simulink model "gm_sampleModel61442_pp_12_1_sub"  (R2023b)
settings: Solver=VariableStepAuto  StartTime=0.0  StopTime=10.0  RelTol=1e-3
libraries: simulink x37
(part 1 of 2)
settings Model: Creator=CW  LastModifiedBy=CW
settings OptimizationCC: BlockReduction=off  ConditionallyExecuteInputs=off
settings DebuggingCC: ArtificialAlgebraicLoopMsg=none  InheritedTsInSrcMsg=none

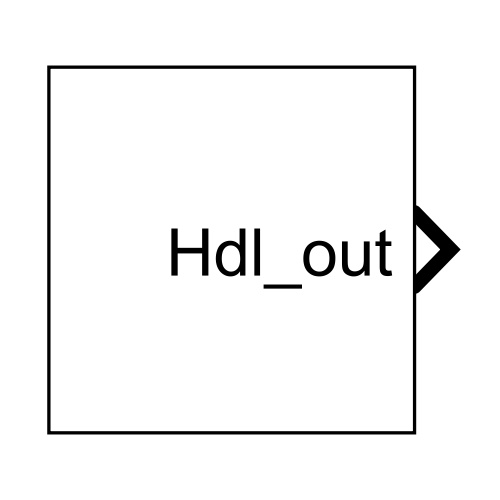
[thumbnail: Simulink's stored preview of the top-level diagram]
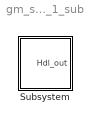
== system gm_sampleModel61442_pp_12_1_sub ==
  Subsystem : Subsystem

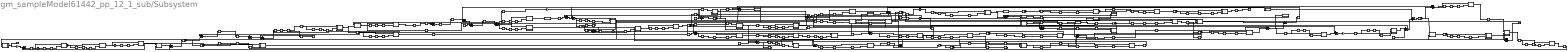
== system gm_sampleModel61442_pp_12_1_sub/Subsystem ==
  Reshape{,1..4} (5 alike) : Reshape
  cfblk1 : Subsystem
  cfblk{10,22,24,46,59,62,66,83,90,93,104} (11 alike) : Sum  Inputs=+  OutDataTypeStr=uint8
  cfblk100 : Subsystem
  cfblk{18,41,50,101} (4 alike) : ComplexToRealImag  SampleTime=1
  cfblk{4..5,14,42,44,57..58,73..74,87,103} (11 alike) : Sum  Inputs=+-  OutDataTypeStr=uint8  AccumDataTypeStr=uint8  SampleTime=1
  cfblk105 : Subsystem
  cfblk106 : Subsystem  mask(Real World Value Increment){}
      mask help: Simulink:masks:RealWorldValueIncrement_MD
      mask Display: disp('V++')
  cfblk108 : Subsystem
  cfblk109 : Subsystem
  cfblk11 : Subsystem
  cfblk110 : Subsystem
  cfblk{26,60,76,96,112} (5 alike) : Gain  Gain="fi(0,0,8,7,\"hex\",\"80\")"  ParamDataTypeStr=fixdt(0, 8, 7)  OutDataTypeStr=uint8  SampleTime=1
  cfblk{68,113,127,129} (4 alike) : MinMax  OutDataTypeStr=uint8
  cfblk{16,27,36,43,51,61,70,82,114..115,118,126,132,142} (14 alike) : Sum  OutDataTypeStr=uint8  AccumDataTypeStr=uint8  SampleTime=1
  cfblk116 : Subsystem
  cfblk{19,30,33,85,117} (5 alike) : Sum  OutDataTypeStr=uint8  AccumDataTypeStr=uint8  RndMeth=Nearest  SampleTime=1
  cfblk117_const_val : Constant  Value=0  VectorParams1D=off  OutDataTypeStr=uint8  SampleTime=1
  cfblk119 : Subsystem
  cfblk{13,35,37,53,64,120,128,138,140} (9 alike) : Abs  SampleTime=1  OutDataTypeStr=uint8  SaturateOnIntegerOverflow=off
  cfblk121 : Subsystem
  cfblk{49,88,99,122,146} (5 alike) : Product  Inputs=*/  OutDataTypeStr=uint8  RndMeth=Zero  SaturateOnIntegerOverflow=on  SampleTime=1
  cfblk{23,39,45,92,98,123,135} (7 alike) : Signum  SampleTime=1
  cfblk124 : Subsystem  mask(Real World Value Increment){}
      mask help: Simulink:masks:RealWorldValueIncrement_MD
      mask Display: disp('V++')
  cfblk125 : Subsystem
  cfblk130_inst : Subsystem
  cfblk134 : Subsystem
  cfblk137 : Subsystem
  cfblk139_inst : Subsystem
  cfblk141_inst : Subsystem
  cfblk143 : Subsystem  mask(Real World Value Increment){}
      mask help: Simulink:masks:RealWorldValueIncrement_MD
      mask Display: disp('V++')
  cfblk144 : Subsystem
  cfblk145 : Subsystem  mask(Real World Value Increment){}
      mask help: Simulink:masks:RealWorldValueIncrement_MD
      mask Display: disp('V++')
  cfblk15 : Subsystem
  cfblk151 : Constant  OutDataTypeStr=uint8  SampleTime=1
  cfblk153 : Subsystem
  cfblk156 : Subsystem
  cfblk157 : Subsystem
  cfblk{158..159,161..167,169..176} (17 alike) : Delay  DelayLength=double(2)  InitialCondition=0  SampleTime=1
  cfblk168 : Subsystem
  cfblk{177..179,182..183,186..187,189..191,193..196} (14 alike) : DataTypeConversion  OutDataTypeStr=fixdt(0,8,0)
  cfblk180 : Subsystem
  cfblk181 : Subsystem
  cfblk184 : Subsystem
  cfblk185 : Subsystem
  cfblk188 : Subsystem
  cfblk192 : Subsystem
  cfblk19_const_val : Constant  Value=0  VectorParams1D=off  OutDataTypeStr=uint8  SampleTime=1
  cfblk2 : Subsystem
  cfblk20 : Subsystem
  cfblk21 : Subsystem
  cfblk25_inst : Subsystem
  cfblk28 : Subsystem
  cfblk3 : Subsystem
  cfblk30_const_val : Constant  Value=0  VectorParams1D=off  OutDataTypeStr=uint8  SampleTime=1
  cfblk31 : Subsystem
  cfblk32 : Subsystem  mask(Real World Value Increment){}
      mask help: Simulink:masks:RealWorldValueIncrement_MD
      mask Display: disp('V++')
  cfblk33_const_val : Constant  Value=0  VectorParams1D=off  OutDataTypeStr=uint8  SampleTime=1
  cfblk40 : Sum  Inputs=+-  OutDataTypeStr=uint8  AccumDataTypeStr=fixdt(1, 32, 7)  SampleTime=1
  cfblk47_inst : Subsystem
  cfblk48 : Subsystem
  cfblk52_inst : Subsystem
  cfblk54_inst : Subsystem
  cfblk71 : Subsystem
  cfblk72 : Subsystem
  cfblk75_inst : Subsystem
  cfblk77 : Subsystem
  cfblk78 : Subsystem
  cfblk79 : Subsystem
  cfblk80 : Subsystem
  cfblk81 : Subsystem
  cfblk84 : Subsystem  mask(Real World Value Increment){}
      mask help: Simulink:masks:RealWorldValueIncrement_MD
      mask Display: disp('V++')
  cfblk85_const_val : Constant  Value=0  VectorParams1D=off  OutDataTypeStr=uint8  SampleTime=1
  cfblk8_inst : Subsystem
  cfblk91 : Subsystem  mask(Real World Value Increment){}
      mask help: Simulink:masks:RealWorldValueIncrement_MD
      mask Display: disp('V++')
  cfblk94_inst : Subsystem
  cfblk97 : Subsystem
  compare{,1,3,7..9,11..15,18..20,22..25,27..28,30,32,35..36} (24 alike) : simulink/Logic and Bit Operations/Compare To Constant  relop=>=  const=0  OutDataTypeStr=boolean
  compare{2,5..6,10,16..17,21,26,29,33} (10 alike) : simulink/Logic and Bit Operations/Compare To Constant  relop=>=  const=255  OutDataTypeStr=boolean
  compare31 : simulink/Logic and Bit Operations/Compare To Constant  relop=>=  const=1  OutDataTypeStr=boolean
  compare34 : simulink/Logic and Bit Operations/Compare To Constant  relop=>=  const=1  OutDataTypeStr=boolean
  compare4 : simulink/Logic and Bit Operations/Compare To Constant  relop=>=  const=1  OutDataTypeStr=boolean
  emi_{6,14,22,30,39,47,55,63,71,79,88,96,104,112,120,128,136,144,152,160,168,176,192,200,208,216,224,232,240,248,256,264,272,281,289,306} (36 alike) : DataTypeConversion  OutDataTypeStr=fixdt(0,8,0)
  emi_{7,23,40,64,89,97,105,113,129,153,161,169,185,193,201,209,233,241,249,265,273,282,290,307} (24 alike) : Delay  DelayLength=double(2)  InitialCondition=0  SampleTime=1
  emi_{31,48,72,121,137,145,177,217,225,257} (10 alike) : Delay  DelayLength=double(2)  InitialCondition=255  SampleTime=1
  emi_15 : Delay  DelayLength=double(2)  InitialCondition=1  SampleTime=1
  emi_184 : DataTypeConversion  OutDataTypeStr=uint8  SampleTime=1  SaturateOnIntegerOverflow=off  RndMeth=Floor
  emi_56 : Delay  DelayLength=double(2)  InitialCondition=1  SampleTime=1
  emi_80 : Delay  DelayLength=double(2)  InitialCondition=1  SampleTime=1
  Hdl_out : Outport  OutDataTypeStr=uint8  SampleTime=1
  wires:
  cfblk1/1(emi_2) -> cfblk60/1, Hdl_out/1
  cfblk10/1 -> emi_129/1, cfblk15/1(emi_123)
  cfblk100/1(emi_10) -> cfblk106/1(u)
  cfblk101/1 -> cfblk146/1
  cfblk101/2 -> cfblk52_inst/1(in1), cfblk187/1
  cfblk103/1 -> cfblk115/2
  cfblk104/1 -> cfblk172/1
  cfblk105/1(emi_18) -> cfblk58/2, cfblk114/1
  cfblk106/1(y) -> cfblk175/1
  cfblk108/1(emi_26) -> emi_225/1, cfblk3/1(emi_219)
  cfblk109/1(emi_34) -> cfblk143/1(u)
  cfblk109/2(emi_35) -> cfblk30/1, cfblk14/1, cfblk170/1
  cfblk11/1(emi_43) -> cfblk101/1
  cfblk110/1(emi_51) -> cfblk40/2
  cfblk112/1 -> cfblk54_inst/2(in2), cfblk10/1
  cfblk113/1 -> cfblk23/1
  cfblk114/1 -> emi_177/1, cfblk21/1(emi_171)
  cfblk115/1 -> cfblk41/1, emi_23/1, cfblk105/1(emi_17)
  cfblk116/1(emi_67) -> cfblk33/1
  cfblk117/1 -> emi_169/1, cfblk171/1, cfblk184/1(emi_163)
  cfblk118/1 -> cfblk179/1
  cfblk119/1(emi_75) -> cfblk195/1
  cfblk120/1 -> cfblk64/1
  cfblk121/1(emi_83) -> cfblk190/1
  cfblk121/2(emi_84) -> cfblk191/1
  cfblk122/1 -> cfblk123/1
  cfblk123/1 -> cfblk18/1
  cfblk124/1(y) -> cfblk70/1
  cfblk125/1(emi_92) -> cfblk193/1
  cfblk126/1 -> cfblk35/1
  cfblk127/1 -> cfblk73/1
  cfblk128/1 -> cfblk92/1
  cfblk129/1 -> cfblk128/1
  cfblk13/1 -> emi_241/1, cfblk134/1(emi_235)
  cfblk130_inst/1(out1) -> emi_257/1, cfblk162/1, cfblk72/1(emi_251)
  cfblk132/1 -> emi_40/1, emi_273/1, cfblk79/1(emi_267), cfblk109/1(emi_33)
  cfblk134/1(emi_236) -> cfblk194/1, cfblk130_inst/2(in2)
  cfblk135/1 -> cfblk19/1, cfblk174/1
  cfblk137/1(emi_108) -> cfblk132/1
  cfblk138/1 -> cfblk173/1
  cfblk139_inst/1(out1) -> cfblk182/1
  cfblk14/1 -> cfblk96/1
  cfblk140/1 -> cfblk90/1
  cfblk141_inst/1(out1) -> cfblk132/2, cfblk103/1
  cfblk142/1 -> cfblk129/1
  cfblk143/1(y) -> cfblk51/2
  cfblk144/1(emi_116) -> cfblk14/2
  cfblk145/1(y) -> Reshape1/1
  cfblk146/1 -> emi_217/1, cfblk20/1(emi_211)
  cfblk15/1(emi_124) -> cfblk146/2, cfblk113/1
  cfblk151/1 -> cfblk44/1
  cfblk153/1(Out1) -> cfblk51/1
  cfblk156/1(Out1) -> cfblk165/1
  cfblk157/1(Out1) -> cfblk84/1(u), cfblk49/1
  cfblk158/1 -> emi_161/1, cfblk181/1(emi_155)
  cfblk159/1 -> cfblk43/2
  cfblk16/1 -> emi_137/1, cfblk78/1(emi_131)
  cfblk161/1 -> cfblk88/1
  cfblk162/1 -> cfblk27/1
  cfblk163/1 -> cfblk61/1
  cfblk164/1 -> cfblk115/1
  cfblk165/1 -> cfblk99/2
  cfblk166/1 -> cfblk57/2
  cfblk167/1 -> emi_7/1, cfblk1/1(emi_1)
  cfblk168/1(emi_59) -> cfblk122/1
  cfblk169/1 -> cfblk47_inst/2(in2)
  cfblk170/1 -> cfblk8_inst/2(in2)
  cfblk171/1 -> cfblk82/2
  cfblk172/1 -> cfblk4/2
  cfblk173/1 -> cfblk49/2
  cfblk174/1 -> cfblk141_inst/1(in1)
  cfblk175/1 -> cfblk103/2
  cfblk176/1 -> cfblk40/1
  cfblk177/1 -> cfblk120/1
  cfblk178/1 -> emi_209/1, cfblk2/1(emi_203)
  cfblk179/1 -> cfblk141_inst/2(in2)
  cfblk18/1 -> cfblk13/1
  cfblk18/2 -> cfblk104/1
  cfblk180/1(emi_148) -> cfblk118/1
  cfblk181/1(emi_156) -> cfblk118/2
  cfblk182/1 -> emi_201/1, cfblk28/1(emi_195)
  cfblk183/1 -> cfblk139_inst/1(in1)
  cfblk184/1(emi_164) -> cfblk139_inst/2(in2)
  cfblk185/1(emi_100) -> emi_307/1, cfblk97/1(emi_300)
  cfblk186/1 -> cfblk36/1
  cfblk187/1 -> cfblk36/2
  cfblk188/1(emi_180) -> emi_249/1, cfblk71/1(emi_243)
  cfblk189/1 -> emi_233/1, cfblk31/1(emi_227)
  cfblk19/1 -> cfblk53/1
  cfblk190/1 -> emi_64/1, cfblk168/1(emi_58)
  cfblk191/1 -> cfblk169/1
  cfblk192/1(emi_188) -> emi_89/1, cfblk121/1(emi_82)
  cfblk193/1 -> cfblk75_inst/2(in2)
  cfblk194/1 -> emi_97/1, cfblk125/1(emi_91)
  cfblk195/1 -> cfblk164/1
  cfblk196/1 -> emi_80/1, cfblk119/1(emi_74)
  cfblk2/1(emi_204) -> cfblk177/1
  cfblk20/1(emi_212) -> cfblk87/2
  cfblk21/1(emi_172) -> cfblk130_inst/1(in1)
  cfblk22/1 -> cfblk27/2
  cfblk23/1 -> cfblk142/1, emi_290/1, cfblk81/1(emi_284)
  cfblk24/1 -> emi_153/1, cfblk180/1(emi_147)
  cfblk25_inst/1(out1) -> cfblk8_inst/1(in1)
  cfblk26/1 -> emi_48/1, cfblk11/1(emi_42)
  cfblk27/1 -> cfblk98/1, emi_56/1, emi_15/1, cfblk100/1(emi_9), cfblk110/1(emi_50)
  cfblk28/1(emi_196) -> cfblk159/1
  cfblk3/1(emi_220) -> cfblk196/1
  cfblk30/1 -> emi_193/1, cfblk192/1(emi_187)
  cfblk31/1(emi_228) -> emi_185/1, cfblk188/1(emi_179)
  cfblk32/1(y) -> cfblk5/1
  cfblk33/1 -> cfblk94_inst/2(in2), cfblk126/2
  cfblk35/1 -> cfblk54_inst/1(in1), cfblk16/2
  cfblk36/1 -> emi_105/1, cfblk185/1(emi_99)
  cfblk37/1 -> cfblk58/1, cfblk16/1
  Reshape/1 -> emi_113/1, cfblk137/1(emi_107)
  cfblk39/1 -> cfblk75_inst/1(in1)
  cfblk4/1 -> cfblk122/2
  cfblk40/1 -> emi_265/1, cfblk77/1(emi_259)
  cfblk41/1 -> Reshape4/1
  cfblk41/2 -> cfblk186/1
  cfblk42/1 -> cfblk166/1
  cfblk43/1 -> cfblk59/1
  cfblk44/1 -> cfblk22/1
  cfblk45/1 -> emi_145/1, cfblk48/1(emi_139)
  cfblk46/1 -> cfblk62/1
  cfblk47_inst/1(out1) -> cfblk43/1
  cfblk48/1(emi_140) -> cfblk70/2, cfblk145/1(u)
  cfblk49/1 -> cfblk26/1
  cfblk5/1 -> cfblk46/1
  cfblk50/1 -> cfblk85/1
  cfblk50/2 -> cfblk138/1, cfblk135/1
  cfblk51/1 -> cfblk99/1
  cfblk52_inst/1(out1) -> cfblk42/1
  cfblk53/1 -> cfblk39/1, cfblk37/1
  cfblk54_inst/1(out1) -> cfblk158/1
  cfblk57/1 -> cfblk44/2
  cfblk58/1 -> cfblk32/1(u)
  cfblk59/1 -> cfblk5/2, cfblk24/1
  cfblk60/1 -> cfblk82/1
  cfblk61/1 -> Reshape2/1
  cfblk62/1 -> cfblk74/1
  Reshape1/1 -> emi_31/1, cfblk108/1(emi_25)
  cfblk64/1 -> cfblk25_inst/2(in2)
  cfblk66/1 -> cfblk57/1
  cfblk68/1 -> emi_72/1, cfblk116/1(emi_66)
  Reshape2/1 -> cfblk66/1
  cfblk70/1 -> cfblk94_inst/1(in1), cfblk52_inst/2(in2), cfblk156/1(In1)
  cfblk71/1(emi_244) -> cfblk47_inst/1(in1)
  cfblk72/1(emi_252) -> cfblk93/1
  cfblk73/1 -> cfblk74/2
  cfblk74/1 -> cfblk4/1
  cfblk75_inst/1(out1) -> Reshape/1, cfblk117/1
  cfblk76/1 -> cfblk88/2
  cfblk77/1(emi_260) -> cfblk112/1, cfblk127/1
  cfblk78/1(emi_132) -> cfblk183/1
  cfblk79/1(emi_268) -> cfblk91/1(u)
  cfblk8_inst/1(out1) -> cfblk73/2, cfblk167/1
  cfblk80/1(emi_276) -> cfblk178/1
  cfblk81/1(emi_285) -> cfblk176/1
  cfblk82/1 -> cfblk189/1
  cfblk83/1 -> emi_121/1, cfblk144/1(emi_115)
  cfblk84/1(y) -> cfblk124/1(u)
  cfblk85/1 -> cfblk25_inst/1(in1), emi_282/1, cfblk80/1(emi_275)
  Reshape3/1 -> cfblk61/2
  cfblk87/1 -> cfblk42/2, cfblk153/1(In1), cfblk83/1
  cfblk88/1 -> cfblk142/2, cfblk157/1(In1)
  cfblk90/1 -> cfblk45/1
  cfblk91/1(y) -> cfblk126/1
  cfblk92/1 -> cfblk87/1
  cfblk93/1 -> cfblk163/1
  cfblk94_inst/1(out1) -> cfblk114/2, cfblk161/1
  Reshape4/1 -> Reshape3/1
  cfblk96/1 -> cfblk68/1
  cfblk97/1(emi_301) -> cfblk50/1
  cfblk98/1 -> cfblk76/1
  cfblk99/1 -> cfblk140/1
  emi_104/1 -> compare/1
  emi_105/1 -> emi_104/1
  emi_112/1 -> compare1/1
  emi_113/1 -> emi_112/1
  emi_120/1 -> compare2/1
  emi_121/1 -> emi_120/1
  emi_128/1 -> compare3/1
  emi_129/1 -> emi_128/1
  emi_136/1 -> compare5/1
  emi_137/1 -> emi_136/1
  emi_14/1 -> compare4/1
  emi_144/1 -> compare6/1
  emi_145/1 -> emi_144/1
  emi_15/1 -> emi_14/1
  emi_152/1 -> compare7/1
  emi_153/1 -> emi_152/1
  emi_160/1 -> compare8/1
  emi_161/1 -> emi_160/1
  emi_168/1 -> compare9/1
  emi_169/1 -> emi_168/1
  emi_176/1 -> compare10/1
  emi_177/1 -> emi_176/1
  emi_184/1 -> compare11/1
  emi_185/1 -> emi_184/1
  emi_192/1 -> compare12/1
  emi_193/1 -> emi_192/1
  emi_200/1 -> compare13/1
  emi_201/1 -> emi_200/1
  emi_208/1 -> compare14/1
  emi_209/1 -> emi_208/1
  emi_216/1 -> compare16/1
  emi_217/1 -> emi_216/1
  emi_22/1 -> compare15/1
  emi_224/1 -> compare17/1
  emi_225/1 -> emi_224/1
  emi_23/1 -> emi_22/1
  emi_232/1 -> compare18/1
  emi_233/1 -> emi_232/1
  emi_240/1 -> compare19/1
  emi_241/1 -> emi_240/1
  emi_248/1 -> compare20/1
  emi_249/1 -> emi_248/1
  emi_256/1 -> compare21/1
  emi_257/1 -> emi_256/1
  emi_264/1 -> compare22/1
  emi_265/1 -> emi_264/1
  emi_272/1 -> compare23/1
  emi_273/1 -> emi_272/1
  emi_281/1 -> compare24/1
  emi_282/1 -> emi_281/1
  emi_289/1 -> compare25/1
  emi_290/1 -> emi_289/1
  emi_30/1 -> compare26/1
  emi_306/1 -> compare27/1
  emi_307/1 -> emi_306/1
  emi_31/1 -> emi_30/1
  emi_39/1 -> compare28/1
  emi_40/1 -> emi_39/1
  emi_47/1 -> compare29/1
  emi_48/1 -> emi_47/1
  emi_55/1 -> compare31/1
  emi_56/1 -> emi_55/1
  emi_6/1 -> compare30/1
  emi_63/1 -> compare32/1
  emi_64/1 -> emi_63/1
  emi_7/1 -> emi_6/1
  emi_71/1 -> compare33/1
  emi_72/1 -> emi_71/1
  emi_79/1 -> compare34/1
  emi_80/1 -> emi_79/1
  emi_88/1 -> compare35/1
  emi_89/1 -> emi_88/1
  emi_96/1 -> compare36/1
  emi_97/1 -> emi_96/1
  cfblk117_const_val/1 -> cfblk117/2
  cfblk19_const_val/1 -> cfblk19/2
  cfblk30_const_val/1 -> cfblk30/2
  cfblk33_const_val/1 -> cfblk33/2
  cfblk85_const_val/1 -> cfblk85/2
  compare/1 -> cfblk185/2(Action Port)
  compare1/1 -> cfblk137/2(Action Port)
  compare2/1 -> cfblk144/2(Action Port)
  compare3/1 -> cfblk15/2(Action Port)
  compare4/1 -> cfblk100/2(Action Port)
  compare5/1 -> cfblk78/2(Action Port)
  compare6/1 -> cfblk48/2(Action Port)
  compare7/1 -> cfblk180/2(Action Port)
  compare8/1 -> cfblk181/2(Action Port)
  compare9/1 -> cfblk184/2(Action Port)
  compare10/1 -> cfblk21/2(Action Port)
  compare11/1 -> cfblk188/2(Action Port)
  compare12/1 -> cfblk192/2(Action Port)
  compare13/1 -> cfblk28/2(Action Port)
  compare14/1 -> cfblk2/2(Action Port)
  compare15/1 -> cfblk105/2(Action Port)
  compare16/1 -> cfblk20/2(Action Port)
  compare17/1 -> cfblk3/2(Action Port)
  compare18/1 -> cfblk31/2(Action Port)
  compare19/1 -> cfblk134/2(Action Port)
  compare20/1 -> cfblk71/2(Action Port)
  compare21/1 -> cfblk72/2(Action Port)
  compare22/1 -> cfblk77/2(Action Port)
  compare23/1 -> cfblk79/2(Action Port)
  compare24/1 -> cfblk80/2(Action Port)
  compare25/1 -> cfblk81/2(Action Port)
  compare26/1 -> cfblk108/2(Action Port)
  compare27/1 -> cfblk97/2(Action Port)
  compare28/1 -> cfblk109/2(Action Port)
  compare29/1 -> cfblk11/2(Action Port)
  compare30/1 -> cfblk1/2(Action Port)
  compare31/1 -> cfblk110/2(Action Port)
  compare32/1 -> cfblk168/2(Action Port)
  compare33/1 -> cfblk116/2(Action Port)
  compare34/1 -> cfblk119/2(Action Port)
  compare35/1 -> cfblk121/2(Action Port)
  compare36/1 -> cfblk125/2(Action Port)

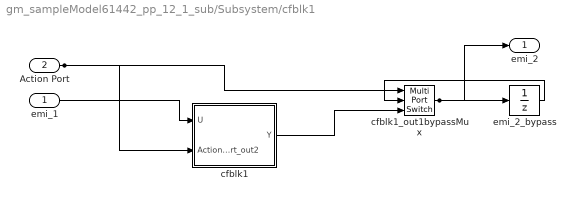
== system gm_sampleModel61442_pp_12_1_sub/Subsystem/cfblk1 ==
  emi_1 : Inport  OutDataTypeStr=uint8  PortDimensions=1  SampleTime=1
  Action Port : Inport  Port=2  OutDataTypeStr=boolean  SampleTime=1
  cfblk1 : Subsystem  mask(Detect Decrease){vinit=double(0), InputProcessing=Elements as channels (sample based), OutDataTypeStr=uint8}
      mask prompts: vinit "Simulink:masks:InitialCondition_MP"; InputProcessing "Simulink:masks:InputProcessing_MP"; OutDataTypeStr "Simulink:masks:OutputDataType_MP"
      mask help: Simulink:masks:DetectDecrease_MD
      mask TypeOptions InputProcessing: Simulink:masks:ColumnsAsChannelsFrameBased | Simulink:masks:ElementsAsChannelsSampleBased
      mask TypeOptions OutDataTypeStr: Simulink:masks:uint8 | Simulink:masks:boolean
      mask Display: fprintf('U < U/z')
  cfblk1_out1bypassMux : MultiPortSwitch  DataPortOrder=Zero-based contiguous  Inputs=2  zeroidx=on  OutDataTypeStr=uint8  SampleTime=1  SaturateOnIntegerOverflow=off  InputSameDT=off
  emi_2_bypass : UnitDelay  InitialCondition="fi(0,0,8,0,\"hex\",\"00\")"  SampleTime=1
  emi_2 : Outport  SampleTime=1  InitialOutput=0
  wires:
  Action Port/1 -> cfblk1_out1bypassMux/1, cfblk1/2(Action Port_out2)
  emi_1/1 -> cfblk1/1(U)
  cfblk1/1(Y) -> cfblk1_out1bypassMux/3
  cfblk1_out1bypassMux/1 -> emi_2_bypass/1, emi_2/1
  emi_2_bypass/1 -> cfblk1_out1bypassMux/2

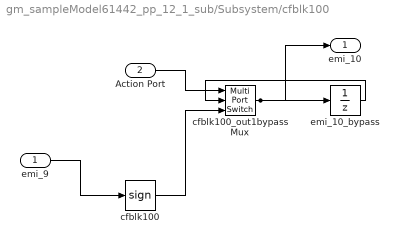
== system gm_sampleModel61442_pp_12_1_sub/Subsystem/cfblk100 ==
  emi_9 : Inport  OutDataTypeStr=uint8  PortDimensions=1  SampleTime=1
  Action Port : Inport  Port=2  OutDataTypeStr=boolean  SampleTime=1
  cfblk100 : Signum  SampleTime=1
  cfblk100_out1bypassMux : MultiPortSwitch  DataPortOrder=Zero-based contiguous  Inputs=2  zeroidx=on  OutDataTypeStr=uint8  SampleTime=1  SaturateOnIntegerOverflow=off  InputSameDT=off
  emi_10_bypass : UnitDelay  InitialCondition="fi(0,0,8,0,\"hex\",\"00\")"  SampleTime=1
  emi_10 : Outport  SampleTime=1  InitialOutput=0
  wires:
  Action Port/1 -> cfblk100_out1bypassMux/1
  emi_9/1 -> cfblk100/1
  cfblk100/1 -> cfblk100_out1bypassMux/3
  cfblk100_out1bypassMux/1 -> emi_10_bypass/1, emi_10/1
  emi_10_bypass/1 -> cfblk100_out1bypassMux/2

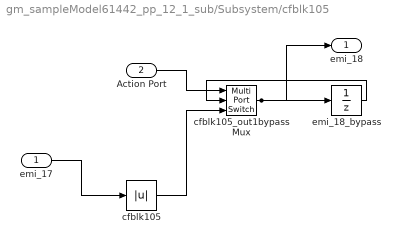
== system gm_sampleModel61442_pp_12_1_sub/Subsystem/cfblk105 ==
  emi_17 : Inport  OutDataTypeStr=uint8  PortDimensions=1  SampleTime=1
  Action Port : Inport  Port=2  OutDataTypeStr=boolean  SampleTime=1
  cfblk105 : Abs  SampleTime=1  OutDataTypeStr=uint8  SaturateOnIntegerOverflow=off
  cfblk105_out1bypassMux : MultiPortSwitch  DataPortOrder=Zero-based contiguous  Inputs=2  zeroidx=on  OutDataTypeStr=uint8  SampleTime=1  SaturateOnIntegerOverflow=off  InputSameDT=off
  emi_18_bypass : UnitDelay  InitialCondition="fi(0,0,8,0,\"hex\",\"00\")"  SampleTime=1
  emi_18 : Outport  SampleTime=1  InitialOutput=0
  wires:
  Action Port/1 -> cfblk105_out1bypassMux/1
  emi_17/1 -> cfblk105/1
  cfblk105/1 -> cfblk105_out1bypassMux/3
  cfblk105_out1bypassMux/1 -> emi_18_bypass/1, emi_18/1
  emi_18_bypass/1 -> cfblk105_out1bypassMux/2

== system gm_sampleModel61442_pp_12_1_sub/Subsystem/cfblk106 ==
  u : Inport  OutDataTypeStr=uint8  SampleTime=1
  FixPt Constant : Constant  DisableCoverage=on  OutDataTypeStr=Inherit: Inherit via back propagation  SampleTime=-1
  FixPt Data Type Duplicate : DataTypeDuplicate  DisableCoverage=on  NumInputPorts=3
  FixPt Sum1 : Sum  OutDataTypeStr=Inherit: Inherit via back propagation  InputSameDT=on  LockScale=on
  y : Outport  SampleTime=1
  wires:
  u/1 -> FixPt Sum1/1, FixPt Data Type Duplicate/2
  FixPt Constant/1 -> FixPt Sum1/2, FixPt Data Type Duplicate/3
  FixPt Sum1/1 -> FixPt Data Type Duplicate/1, y/1

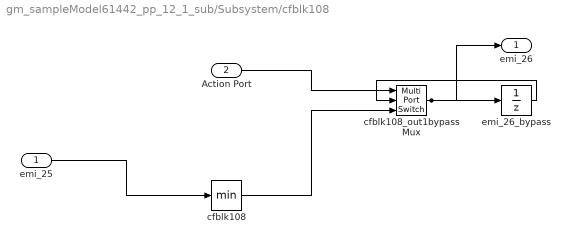
== system gm_sampleModel61442_pp_12_1_sub/Subsystem/cfblk108 ==
  emi_25 : Inport  OutDataTypeStr=uint8  PortDimensions=1  SampleTime=1
  Action Port : Inport  Port=2  OutDataTypeStr=boolean  SampleTime=1
  cfblk108 : MinMax
  cfblk108_out1bypassMux : MultiPortSwitch  DataPortOrder=Zero-based contiguous  Inputs=2  zeroidx=on  OutDataTypeStr=uint8  SampleTime=1  SaturateOnIntegerOverflow=off  InputSameDT=off
  emi_26_bypass : UnitDelay  InitialCondition="fi(0,0,8,0,\"hex\",\"00\")"  SampleTime=1
  emi_26 : Outport  SampleTime=1  InitialOutput=0
  wires:
  Action Port/1 -> cfblk108_out1bypassMux/1
  emi_25/1 -> cfblk108/1
  cfblk108/1 -> cfblk108_out1bypassMux/3
  cfblk108_out1bypassMux/1 -> emi_26_bypass/1, emi_26/1
  emi_26_bypass/1 -> cfblk108_out1bypassMux/2

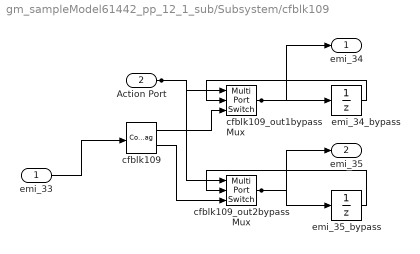
== system gm_sampleModel61442_pp_12_1_sub/Subsystem/cfblk109 ==
  emi_33 : Inport  OutDataTypeStr=uint8  PortDimensions=1  SampleTime=1
  Action Port : Inport  Port=2  OutDataTypeStr=boolean  SampleTime=1
  cfblk109 : ComplexToRealImag  SampleTime=1
  cfblk109_out1bypassMux : MultiPortSwitch  DataPortOrder=Zero-based contiguous  Inputs=2  zeroidx=on  OutDataTypeStr=uint8  SampleTime=1  SaturateOnIntegerOverflow=off  InputSameDT=off
  cfblk109_out2bypassMux : MultiPortSwitch  DataPortOrder=Zero-based contiguous  Inputs=2  zeroidx=on  OutDataTypeStr=uint8  SampleTime=1  SaturateOnIntegerOverflow=off  InputSameDT=off
  emi_34_bypass : UnitDelay  InitialCondition="fi(0,0,8,0,\"hex\",\"00\")"  SampleTime=1
  emi_35_bypass : UnitDelay  InitialCondition="fi(0,0,8,0,\"hex\",\"00\")"  SampleTime=1
  emi_34 : Outport  SampleTime=1  InitialOutput=0
  emi_35 : Outport  Port=2  SampleTime=1  InitialOutput=0
  wires:
  Action Port/1 -> cfblk109_out2bypassMux/1, cfblk109_out1bypassMux/1
  emi_33/1 -> cfblk109/1
  cfblk109/1 -> cfblk109_out1bypassMux/3
  cfblk109/2 -> cfblk109_out2bypassMux/3
  cfblk109_out1bypassMux/1 -> emi_34_bypass/1, emi_34/1
  emi_34_bypass/1 -> cfblk109_out1bypassMux/2
  cfblk109_out2bypassMux/1 -> emi_35_bypass/1, emi_35/1
  emi_35_bypass/1 -> cfblk109_out2bypassMux/2

== system gm_sampleModel61442_pp_12_1_sub/Subsystem/cfblk11 ==
  emi_42 : Inport  OutDataTypeStr=uint8  PortDimensions=1  SampleTime=1
  Action Port : Inport  Port=2  OutDataTypeStr=boolean  SampleTime=1
  cfblk11 : MinMax
  cfblk11_out1bypassMux : MultiPortSwitch  DataPortOrder=Zero-based contiguous  Inputs=2  zeroidx=on  OutDataTypeStr=uint8  SampleTime=1  SaturateOnIntegerOverflow=off  InputSameDT=off
  emi_43_bypass : UnitDelay  InitialCondition="fi(0,0,8,0,\"hex\",\"00\")"  SampleTime=1
  emi_43 : Outport  SampleTime=1  InitialOutput=0
  wires:
  Action Port/1 -> cfblk11_out1bypassMux/1
  emi_42/1 -> cfblk11/1
  cfblk11/1 -> cfblk11_out1bypassMux/3
  cfblk11_out1bypassMux/1 -> emi_43_bypass/1, emi_43/1
  emi_43_bypass/1 -> cfblk11_out1bypassMux/2

== system gm_sampleModel61442_pp_12_1_sub/Subsystem/cfblk110 ==
  emi_50 : Inport  OutDataTypeStr=uint8  PortDimensions=1  SampleTime=1
  Action Port : Inport  Port=2  OutDataTypeStr=boolean  SampleTime=1
  cfblk110 : Gain  Gain="fi(0,0,8,7,\"hex\",\"80\")"  ParamDataTypeStr=fixdt(0, 8, 7)  OutDataTypeStr=fixdt(0, 16, 7)  SampleTime=1
  cfblk110_out1bypassMux : MultiPortSwitch  DataPortOrder=Zero-based contiguous  Inputs=2  zeroidx=on  OutDataTypeStr=fixdt(0, 16, 7)  SampleTime=1  SaturateOnIntegerOverflow=off  InputSameDT=off
  emi_51_bypass : UnitDelay  InitialCondition="fi(0,0,16,7,\"hex\",\"0000\")"  SampleTime=1
  emi_51 : Outport  SampleTime=1  InitialOutput=0
  wires:
  Action Port/1 -> cfblk110_out1bypassMux/1
  emi_50/1 -> cfblk110/1
  cfblk110/1 -> cfblk110_out1bypassMux/3
  cfblk110_out1bypassMux/1 -> emi_51_bypass/1, emi_51/1
  emi_51_bypass/1 -> cfblk110_out1bypassMux/2

== system gm_sampleModel61442_pp_12_1_sub/Subsystem/cfblk116 ==
  emi_66 : Inport  OutDataTypeStr=uint8  PortDimensions=1  SampleTime=1
  Action Port : Inport  Port=2  OutDataTypeStr=boolean  SampleTime=1
  cfblk116 : Abs  SampleTime=1  OutDataTypeStr=uint8  SaturateOnIntegerOverflow=off
  cfblk116_out1bypassMux : MultiPortSwitch  DataPortOrder=Zero-based contiguous  Inputs=2  zeroidx=on  OutDataTypeStr=uint8  SampleTime=1  SaturateOnIntegerOverflow=off  InputSameDT=off
  emi_67_bypass : UnitDelay  InitialCondition="fi(0,0,8,0,\"hex\",\"00\")"  SampleTime=1
  emi_67 : Outport  SampleTime=1  InitialOutput=0
  wires:
  Action Port/1 -> cfblk116_out1bypassMux/1
  emi_66/1 -> cfblk116/1
  cfblk116/1 -> cfblk116_out1bypassMux/3
  cfblk116_out1bypassMux/1 -> emi_67_bypass/1, emi_67/1
  emi_67_bypass/1 -> cfblk116_out1bypassMux/2

== system gm_sampleModel61442_pp_12_1_sub/Subsystem/cfblk119 ==
  emi_74 : Inport  OutDataTypeStr=uint8  PortDimensions=1  SampleTime=1
  Action Port : Inport  Port=2  OutDataTypeStr=boolean  SampleTime=1
  cfblk119 : Subsystem  mask(Real World Value Increment){}
      mask help: Simulink:masks:RealWorldValueIncrement_MD
      mask Display: disp('V++')
  cfblk119_out1bypassMux : MultiPortSwitch  DataPortOrder=Zero-based contiguous  Inputs=2  zeroidx=on  OutDataTypeStr=uint8  SampleTime=1  SaturateOnIntegerOverflow=off  InputSameDT=off
  emi_75_bypass : UnitDelay  InitialCondition="fi(0,0,8,0,\"hex\",\"00\")"  SampleTime=1
  emi_75 : Outport  SampleTime=1  InitialOutput=0
  wires:
  Action Port/1 -> cfblk119_out1bypassMux/1
  emi_74/1 -> cfblk119/1(u)
  cfblk119/1(y) -> cfblk119_out1bypassMux/3
  cfblk119_out1bypassMux/1 -> emi_75_bypass/1, emi_75/1
  emi_75_bypass/1 -> cfblk119_out1bypassMux/2

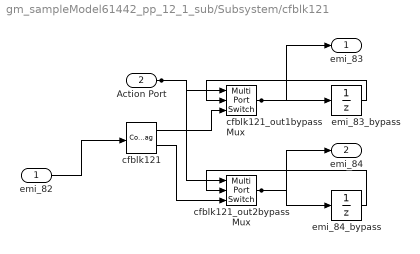
== system gm_sampleModel61442_pp_12_1_sub/Subsystem/cfblk121 ==
  emi_82 : Inport  OutDataTypeStr=uint8  PortDimensions=1  SampleTime=1
  Action Port : Inport  Port=2  OutDataTypeStr=boolean  SampleTime=1
  cfblk121 : ComplexToRealImag  SampleTime=1
  cfblk121_out1bypassMux : MultiPortSwitch  DataPortOrder=Zero-based contiguous  Inputs=2  zeroidx=on  OutDataTypeStr=uint8  SampleTime=1  SaturateOnIntegerOverflow=off  InputSameDT=off
  cfblk121_out2bypassMux : MultiPortSwitch  DataPortOrder=Zero-based contiguous  Inputs=2  zeroidx=on  OutDataTypeStr=uint8  SampleTime=1  SaturateOnIntegerOverflow=off  InputSameDT=off
  emi_83_bypass : UnitDelay  InitialCondition="fi(0,0,8,0,\"hex\",\"00\")"  SampleTime=1
  emi_84_bypass : UnitDelay  InitialCondition="fi(0,0,8,0,\"hex\",\"00\")"  SampleTime=1
  emi_83 : Outport  SampleTime=1  InitialOutput=0
  emi_84 : Outport  Port=2  SampleTime=1  InitialOutput=0
  wires:
  Action Port/1 -> cfblk121_out2bypassMux/1, cfblk121_out1bypassMux/1
  emi_82/1 -> cfblk121/1
  cfblk121/1 -> cfblk121_out1bypassMux/3
  cfblk121/2 -> cfblk121_out2bypassMux/3
  cfblk121_out1bypassMux/1 -> emi_83_bypass/1, emi_83/1
  emi_83_bypass/1 -> cfblk121_out1bypassMux/2
  cfblk121_out2bypassMux/1 -> emi_84_bypass/1, emi_84/1
  emi_84_bypass/1 -> cfblk121_out2bypassMux/2

== system gm_sampleModel61442_pp_12_1_sub/Subsystem/cfblk124 ==
  u : Inport  OutDataTypeStr=uint8  SampleTime=1
  FixPt Constant : Constant  DisableCoverage=on  OutDataTypeStr=Inherit: Inherit via back propagation  SampleTime=-1
  FixPt Data Type Duplicate : DataTypeDuplicate  DisableCoverage=on  NumInputPorts=3
  FixPt Sum1 : Sum  OutDataTypeStr=Inherit: Inherit via back propagation  InputSameDT=on  LockScale=on
  y : Outport  SampleTime=1
  wires:
  u/1 -> FixPt Sum1/1, FixPt Data Type Duplicate/2
  FixPt Constant/1 -> FixPt Sum1/2, FixPt Data Type Duplicate/3
  FixPt Sum1/1 -> FixPt Data Type Duplicate/1, y/1

== system gm_sampleModel61442_pp_12_1_sub/Subsystem/cfblk125 ==
  emi_91 : Inport  OutDataTypeStr=uint8  PortDimensions=1  SampleTime=1
  Action Port : Inport  Port=2  OutDataTypeStr=boolean  SampleTime=1
  cfblk125 : MinMax
  cfblk125_out1bypassMux : MultiPortSwitch  DataPortOrder=Zero-based contiguous  Inputs=2  zeroidx=on  OutDataTypeStr=uint8  SampleTime=1  SaturateOnIntegerOverflow=off  InputSameDT=off
  emi_92_bypass : UnitDelay  InitialCondition="fi(0,0,8,0,\"hex\",\"00\")"  SampleTime=1
  emi_92 : Outport  SampleTime=1  InitialOutput=0
  wires:
  Action Port/1 -> cfblk125_out1bypassMux/1
  emi_91/1 -> cfblk125/1
  cfblk125/1 -> cfblk125_out1bypassMux/3
  cfblk125_out1bypassMux/1 -> emi_92_bypass/1, emi_92/1
  emi_92_bypass/1 -> cfblk125_out1bypassMux/2

== system gm_sampleModel61442_pp_12_1_sub/Subsystem/cfblk130_inst ==
  in1 : Inport  OutDataTypeStr=uint8  SampleTime=1
  in2 : Inport  Port=2  OutDataTypeStr=uint8  SampleTime=1
  mul_cfblk130_dotp_mulcomp : Product  Inputs=**  OutDataTypeStr=uint8  SampleTime=1
  out1 : Outport  OutDataTypeStr=uint8  SampleTime=1
  wires:
  in1/1 -> mul_cfblk130_dotp_mulcomp/1
  in2/1 -> mul_cfblk130_dotp_mulcomp/2
  mul_cfblk130_dotp_mulcomp/1 -> out1/1

== system gm_sampleModel61442_pp_12_1_sub/Subsystem/cfblk134 ==
  emi_235 : Inport  OutDataTypeStr=uint8  PortDimensions=1  SampleTime=1
  Action Port : Inport  Port=2  OutDataTypeStr=boolean  SampleTime=1
  Reshape : Reshape
  cfblk134_out1bypassMux : MultiPortSwitch  DataPortOrder=Zero-based contiguous  Inputs=2  zeroidx=on  OutDataTypeStr=uint8  SampleTime=1  SaturateOnIntegerOverflow=off  InputSameDT=off
  emi_236_bypass : UnitDelay  InitialCondition="fi(0,0,8,0,\"hex\",\"00\")"  SampleTime=1
  emi_236 : Outport  SampleTime=1  InitialOutput=0
  wires:
  Action Port/1 -> cfblk134_out1bypassMux/1
  emi_235/1 -> Reshape/1
  Reshape/1 -> cfblk134_out1bypassMux/3
  cfblk134_out1bypassMux/1 -> emi_236_bypass/1, emi_236/1
  emi_236_bypass/1 -> cfblk134_out1bypassMux/2

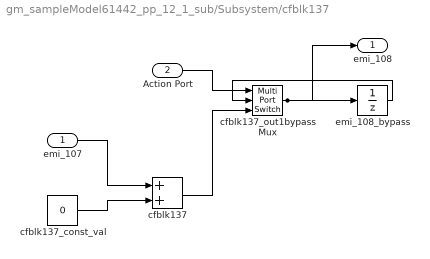
== system gm_sampleModel61442_pp_12_1_sub/Subsystem/cfblk137 ==
  emi_107 : Inport  OutDataTypeStr=uint8  PortDimensions=1  SampleTime=1
  Action Port : Inport  Port=2  OutDataTypeStr=boolean  SampleTime=1
  cfblk137 : Sum  OutDataTypeStr=uint8  AccumDataTypeStr=uint8  RndMeth=Nearest  SampleTime=1
  cfblk137_const_val : Constant  Value=0  VectorParams1D=off  OutDataTypeStr=uint8  SampleTime=1
  cfblk137_out1bypassMux : MultiPortSwitch  DataPortOrder=Zero-based contiguous  Inputs=2  zeroidx=on  OutDataTypeStr=uint8  SampleTime=1  SaturateOnIntegerOverflow=off  InputSameDT=off
  emi_108_bypass : UnitDelay  InitialCondition="fi(0,0,8,0,\"hex\",\"00\")"  SampleTime=1
  emi_108 : Outport  SampleTime=1  InitialOutput=0
  wires:
  Action Port/1 -> cfblk137_out1bypassMux/1
  emi_107/1 -> cfblk137/1
  cfblk137/1 -> cfblk137_out1bypassMux/3
  cfblk137_out1bypassMux/1 -> emi_108_bypass/1, emi_108/1
  emi_108_bypass/1 -> cfblk137_out1bypassMux/2
  cfblk137_const_val/1 -> cfblk137/2

== system gm_sampleModel61442_pp_12_1_sub/Subsystem/cfblk139_inst ==
  in1 : Inport  OutDataTypeStr=uint8  SampleTime=1
  in2 : Inport  Port=2  OutDataTypeStr=uint8  SampleTime=1
  mul_cfblk139_dotp_mulcomp : Product  Inputs=**  OutDataTypeStr=uint8  SampleTime=1
  out1 : Outport  OutDataTypeStr=uint8  SampleTime=1
  wires:
  in1/1 -> mul_cfblk139_dotp_mulcomp/1
  in2/1 -> mul_cfblk139_dotp_mulcomp/2
  mul_cfblk139_dotp_mulcomp/1 -> out1/1

== system gm_sampleModel61442_pp_12_1_sub/Subsystem/cfblk141_inst ==
  in1 : Inport  OutDataTypeStr=uint8  SampleTime=1
  in2 : Inport  Port=2  OutDataTypeStr=uint8  SampleTime=1
  mul_cfblk141_dotp_mulcomp : Product  Inputs=**  OutDataTypeStr=uint8  SampleTime=1
  out1 : Outport  OutDataTypeStr=uint8  SampleTime=1
  wires:
  in1/1 -> mul_cfblk141_dotp_mulcomp/1
  in2/1 -> mul_cfblk141_dotp_mulcomp/2
  mul_cfblk141_dotp_mulcomp/1 -> out1/1

== system gm_sampleModel61442_pp_12_1_sub/Subsystem/cfblk143 ==
  u : Inport  OutDataTypeStr=uint8  SampleTime=1
  FixPt Constant : Constant  DisableCoverage=on  OutDataTypeStr=Inherit: Inherit via back propagation  SampleTime=-1
  FixPt Data Type Duplicate : DataTypeDuplicate  DisableCoverage=on  NumInputPorts=3
  FixPt Sum1 : Sum  OutDataTypeStr=Inherit: Inherit via back propagation  InputSameDT=on  LockScale=on
  y : Outport  SampleTime=1
  wires:
  u/1 -> FixPt Sum1/1, FixPt Data Type Duplicate/2
  FixPt Constant/1 -> FixPt Sum1/2, FixPt Data Type Duplicate/3
  FixPt Sum1/1 -> FixPt Data Type Duplicate/1, y/1

== system gm_sampleModel61442_pp_12_1_sub/Subsystem/cfblk144 ==
  emi_115 : Inport  OutDataTypeStr=uint8  PortDimensions=1  SampleTime=1
  Action Port : Inport  Port=2  OutDataTypeStr=boolean  SampleTime=1
  Reshape : Reshape
  cfblk144_out1bypassMux : MultiPortSwitch  DataPortOrder=Zero-based contiguous  Inputs=2  zeroidx=on  OutDataTypeStr=uint8  SampleTime=1  SaturateOnIntegerOverflow=off  InputSameDT=off
  emi_116_bypass : UnitDelay  InitialCondition="fi(0,0,8,0,\"hex\",\"00\")"  SampleTime=1
  emi_116 : Outport  SampleTime=1  InitialOutput=0
  wires:
  Action Port/1 -> cfblk144_out1bypassMux/1
  emi_115/1 -> Reshape/1
  Reshape/1 -> cfblk144_out1bypassMux/3
  cfblk144_out1bypassMux/1 -> emi_116_bypass/1, emi_116/1
  emi_116_bypass/1 -> cfblk144_out1bypassMux/2

== system gm_sampleModel61442_pp_12_1_sub/Subsystem/cfblk145 ==
  u : Inport  OutDataTypeStr=uint8  SampleTime=1
  FixPt Constant : Constant  DisableCoverage=on  OutDataTypeStr=Inherit: Inherit via back propagation  SampleTime=-1
  FixPt Data Type Duplicate : DataTypeDuplicate  DisableCoverage=on  NumInputPorts=3
  FixPt Sum1 : Sum  OutDataTypeStr=Inherit: Inherit via back propagation  InputSameDT=on  LockScale=on
  y : Outport  SampleTime=1
  wires:
  u/1 -> FixPt Sum1/1, FixPt Data Type Duplicate/2
  FixPt Constant/1 -> FixPt Sum1/2, FixPt Data Type Duplicate/3
  FixPt Sum1/1 -> FixPt Data Type Duplicate/1, y/1

== system gm_sampleModel61442_pp_12_1_sub/Subsystem/cfblk15 ==
  emi_123 : Inport  OutDataTypeStr=uint8  PortDimensions=1  SampleTime=1
  Action Port : Inport  Port=2  OutDataTypeStr=boolean  SampleTime=1
  cfblk15 : MinMax
  cfblk15_out1bypassMux : MultiPortSwitch  DataPortOrder=Zero-based contiguous  Inputs=2  zeroidx=on  OutDataTypeStr=uint8  SampleTime=1  SaturateOnIntegerOverflow=off  InputSameDT=off
  emi_124_bypass : UnitDelay  InitialCondition="fi(0,0,8,0,\"hex\",\"00\")"  SampleTime=1
  emi_124 : Outport  SampleTime=1  InitialOutput=0
  wires:
  Action Port/1 -> cfblk15_out1bypassMux/1
  emi_123/1 -> cfblk15/1
  cfblk15/1 -> cfblk15_out1bypassMux/3
  cfblk15_out1bypassMux/1 -> emi_124_bypass/1, emi_124/1
  emi_124_bypass/1 -> cfblk15_out1bypassMux/2

== system gm_sampleModel61442_pp_12_1_sub/Subsystem/cfblk153 ==
  In1 : Inport  OutDataTypeStr=uint8  PortDimensions=1  SampleTime=1
  Out1 : Outport  SampleTime=1  InitialOutput=[0]
  wires:
  In1/1 -> Out1/1

== system gm_sampleModel61442_pp_12_1_sub/Subsystem/cfblk156 ==
  In1 : Inport  OutDataTypeStr=uint8  PortDimensions=1  SampleTime=1
  Out1 : Outport  SampleTime=1  InitialOutput=[0]
  wires:
  In1/1 -> Out1/1

== system gm_sampleModel61442_pp_12_1_sub/Subsystem/cfblk157 ==
  In1 : Inport  OutDataTypeStr=uint8  PortDimensions=1  SampleTime=1
  Out1 : Outport  SampleTime=1  InitialOutput=[0]
  wires:
  In1/1 -> Out1/1

== system gm_sampleModel61442_pp_12_1_sub/Subsystem/cfblk168 ==
  emi_58 : Inport  OutDataTypeStr=uint8  PortDimensions=1  SampleTime=1
  Action Port : Inport  Port=2  OutDataTypeStr=boolean  SampleTime=1
  cfblk168 : Subsystem
      settings: MinAlgLoopOccurrences=on
  emi_59 : Outport  SampleTime=1  InitialOutput=0
  wires:
  Action Port/1 -> cfblk168/Enable
  emi_58/1 -> cfblk168/1(in0)
  cfblk168/1(out0) -> emi_59/1

== system gm_sampleModel61442_pp_12_1_sub/Subsystem/cfblk180 ==
  emi_147 : Inport  OutDataTypeStr=uint8  PortDimensions=1  SampleTime=1
  Action Port : Inport  Port=2  OutDataTypeStr=boolean  SampleTime=1
  cfblk180 : DataTypeConversion  OutDataTypeStr=fixdt(0,8,0)
  cfblk180_out1bypassMux : MultiPortSwitch  DataPortOrder=Zero-based contiguous  Inputs=2  zeroidx=on  OutDataTypeStr=uint8  SampleTime=1  SaturateOnIntegerOverflow=off  InputSameDT=off
  emi_148_bypass : UnitDelay  InitialCondition="fi(0,0,8,0,\"hex\",\"00\")"  SampleTime=1
  emi_148 : Outport  SampleTime=1  InitialOutput=0
  wires:
  Action Port/1 -> cfblk180_out1bypassMux/1
  emi_147/1 -> cfblk180/1
  cfblk180/1 -> cfblk180_out1bypassMux/3
  cfblk180_out1bypassMux/1 -> emi_148_bypass/1, emi_148/1
  emi_148_bypass/1 -> cfblk180_out1bypassMux/2

== system gm_sampleModel61442_pp_12_1_sub/Subsystem/cfblk181 ==
  emi_155 : Inport  OutDataTypeStr=uint8  PortDimensions=1  SampleTime=1
  Action Port : Inport  Port=2  OutDataTypeStr=boolean  SampleTime=1
  cfblk181 : DataTypeConversion  OutDataTypeStr=fixdt(0,8,0)
  cfblk181_out1bypassMux : MultiPortSwitch  DataPortOrder=Zero-based contiguous  Inputs=2  zeroidx=on  OutDataTypeStr=uint8  SampleTime=1  SaturateOnIntegerOverflow=off  InputSameDT=off
  emi_156_bypass : UnitDelay  InitialCondition="fi(0,0,8,0,\"hex\",\"00\")"  SampleTime=1
  emi_156 : Outport  SampleTime=1  InitialOutput=0
  wires:
  Action Port/1 -> cfblk181_out1bypassMux/1
  emi_155/1 -> cfblk181/1
  cfblk181/1 -> cfblk181_out1bypassMux/3
  cfblk181_out1bypassMux/1 -> emi_156_bypass/1, emi_156/1
  emi_156_bypass/1 -> cfblk181_out1bypassMux/2

== system gm_sampleModel61442_pp_12_1_sub/Subsystem/cfblk184 ==
  emi_163 : Inport  OutDataTypeStr=uint8  PortDimensions=1  SampleTime=1
  Action Port : Inport  Port=2  OutDataTypeStr=boolean  SampleTime=1
  cfblk184 : DataTypeConversion  OutDataTypeStr=fixdt(0,8,0)
  cfblk184_out1bypassMux : MultiPortSwitch  DataPortOrder=Zero-based contiguous  Inputs=2  zeroidx=on  OutDataTypeStr=uint8  SampleTime=1  SaturateOnIntegerOverflow=off  InputSameDT=off
  emi_164_bypass : UnitDelay  InitialCondition="fi(0,0,8,0,\"hex\",\"00\")"  SampleTime=1
  emi_164 : Outport  SampleTime=1  InitialOutput=0
  wires:
  Action Port/1 -> cfblk184_out1bypassMux/1
  emi_163/1 -> cfblk184/1
  cfblk184/1 -> cfblk184_out1bypassMux/3
  cfblk184_out1bypassMux/1 -> emi_164_bypass/1, emi_164/1
  emi_164_bypass/1 -> cfblk184_out1bypassMux/2

== system gm_sampleModel61442_pp_12_1_sub/Subsystem/cfblk185 ==
  emi_99 : Inport  OutDataTypeStr=uint8  PortDimensions=1  SampleTime=1
  Action Port : Inport  Port=2  OutDataTypeStr=boolean  SampleTime=1
  cfblk185 : DataTypeConversion  OutDataTypeStr=fixdt(0,8,0)
  cfblk185_out1bypassMux : MultiPortSwitch  DataPortOrder=Zero-based contiguous  Inputs=2  zeroidx=on  OutDataTypeStr=uint8  SampleTime=1  SaturateOnIntegerOverflow=off  InputSameDT=off
  emi_100_bypass : UnitDelay  InitialCondition="fi(0,0,8,0,\"hex\",\"00\")"  SampleTime=1
  emi_100 : Outport  SampleTime=1  InitialOutput=0
  wires:
  Action Port/1 -> cfblk185_out1bypassMux/1
  emi_99/1 -> cfblk185/1
  cfblk185/1 -> cfblk185_out1bypassMux/3
  cfblk185_out1bypassMux/1 -> emi_100_bypass/1, emi_100/1
  emi_100_bypass/1 -> cfblk185_out1bypassMux/2

== system gm_sampleModel61442_pp_12_1_sub/Subsystem/cfblk188 ==
  emi_179 : Inport  OutDataTypeStr=fixdt(0, 16, 7)  PortDimensions=1  SampleTime=1
  Action Port : Inport  Port=2  OutDataTypeStr=boolean  SampleTime=1
  cfblk188 : DataTypeConversion  OutDataTypeStr=uint8  SampleTime=1  SaturateOnIntegerOverflow=off  RndMeth=Floor
  cfblk188_out1bypassMux : MultiPortSwitch  DataPortOrder=Zero-based contiguous  Inputs=2  zeroidx=on  OutDataTypeStr=uint8  SampleTime=1  SaturateOnIntegerOverflow=off  InputSameDT=off
  emi_180_bypass : UnitDelay  InitialCondition="fi(0,0,8,0,\"hex\",\"00\")"  SampleTime=1
  emi_180 : Outport  SampleTime=1  InitialOutput=0
  wires:
  Action Port/1 -> cfblk188_out1bypassMux/1
  emi_179/1 -> cfblk188/1
  cfblk188/1 -> cfblk188_out1bypassMux/3
  cfblk188_out1bypassMux/1 -> emi_180_bypass/1, emi_180/1
  emi_180_bypass/1 -> cfblk188_out1bypassMux/2

== system gm_sampleModel61442_pp_12_1_sub/Subsystem/cfblk192 ==
  emi_187 : Inport  OutDataTypeStr=uint8  PortDimensions=1  SampleTime=1
  Action Port : Inport  Port=2  OutDataTypeStr=boolean  SampleTime=1
  cfblk192 : DataTypeConversion  OutDataTypeStr=fixdt(0,8,0)
  cfblk192_out1bypassMux : MultiPortSwitch  DataPortOrder=Zero-based contiguous  Inputs=2  zeroidx=on  OutDataTypeStr=uint8  SampleTime=1  SaturateOnIntegerOverflow=off  InputSameDT=off
  emi_188_bypass : UnitDelay  InitialCondition="fi(0,0,8,0,\"hex\",\"00\")"  SampleTime=1
  emi_188 : Outport  SampleTime=1  InitialOutput=0
  wires:
  Action Port/1 -> cfblk192_out1bypassMux/1
  emi_187/1 -> cfblk192/1
  cfblk192/1 -> cfblk192_out1bypassMux/3
  cfblk192_out1bypassMux/1 -> emi_188_bypass/1, emi_188/1
  emi_188_bypass/1 -> cfblk192_out1bypassMux/2

== system gm_sampleModel61442_pp_12_1_sub/Subsystem/cfblk2 ==
  emi_203 : Inport  OutDataTypeStr=uint8  PortDimensions=1  SampleTime=1
  Action Port : Inport  Port=2  OutDataTypeStr=boolean  SampleTime=1
  cfblk2 : Subsystem  mask(Detect Rise Positive){vinit=double(0), InputProcessing=Elements as channels (sample based), OutDataTypeStr=uint8}
      mask prompts: vinit "Simulink:masks:InitialCondition_MP"; InputProcessing "Simulink:masks:InputProcessing_MP"; OutDataTypeStr "Simulink:masks:OutputDataType_MP"
      mask help: Simulink:masks:DetectRisePositive_MD
      mask TypeOptions InputProcessing: Simulink:masks:ColumnsAsChannelsFrameBased | Simulink:masks:ElementsAsChannelsSampleBased
      mask TypeOptions OutDataTypeStr: Simulink:masks:uint8 | Simulink:masks:boolean
      mask Display: fprintf('U > 0\n&  NOT\nU/z > 0')
  cfblk2_out1bypassMux : MultiPortSwitch  DataPortOrder=Zero-based contiguous  Inputs=2  zeroidx=on  OutDataTypeStr=uint8  SampleTime=1  SaturateOnIntegerOverflow=off  InputSameDT=off
  emi_204_bypass : UnitDelay  InitialCondition="fi(0,0,8,0,\"hex\",\"00\")"  SampleTime=1
  emi_204 : Outport  SampleTime=1  InitialOutput=0
  wires:
  Action Port/1 -> cfblk2_out1bypassMux/1, cfblk2/2(Action Port_out2)
  emi_203/1 -> cfblk2/1(U)
  cfblk2/1(Y) -> cfblk2_out1bypassMux/3
  cfblk2_out1bypassMux/1 -> emi_204_bypass/1, emi_204/1
  emi_204_bypass/1 -> cfblk2_out1bypassMux/2

== system gm_sampleModel61442_pp_12_1_sub/Subsystem/cfblk20 ==
  emi_211 : Inport  OutDataTypeStr=uint8  PortDimensions=1  SampleTime=1
  Action Port : Inport  Port=2  OutDataTypeStr=boolean  SampleTime=1
  cfblk20 : Signum  SampleTime=1
  cfblk20_out1bypassMux : MultiPortSwitch  DataPortOrder=Zero-based contiguous  Inputs=2  zeroidx=on  OutDataTypeStr=uint8  SampleTime=1  SaturateOnIntegerOverflow=off  InputSameDT=off
  emi_212_bypass : UnitDelay  InitialCondition="fi(0,0,8,0,\"hex\",\"00\")"  SampleTime=1
  emi_212 : Outport  SampleTime=1  InitialOutput=0
  wires:
  Action Port/1 -> cfblk20_out1bypassMux/1
  emi_211/1 -> cfblk20/1
  cfblk20/1 -> cfblk20_out1bypassMux/3
  cfblk20_out1bypassMux/1 -> emi_212_bypass/1, emi_212/1
  emi_212_bypass/1 -> cfblk20_out1bypassMux/2

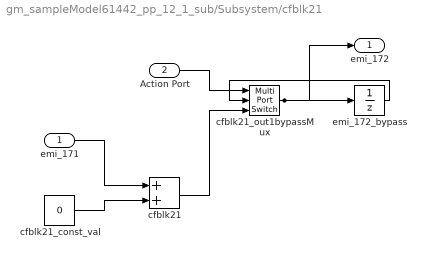
== system gm_sampleModel61442_pp_12_1_sub/Subsystem/cfblk21 ==
  emi_171 : Inport  OutDataTypeStr=uint8  PortDimensions=1  SampleTime=1
  Action Port : Inport  Port=2  OutDataTypeStr=boolean  SampleTime=1
  cfblk21 : Sum  OutDataTypeStr=uint8  AccumDataTypeStr=uint8  RndMeth=Nearest  SampleTime=1
  cfblk21_const_val : Constant  Value=0  VectorParams1D=off  OutDataTypeStr=uint8  SampleTime=1
  cfblk21_out1bypassMux : MultiPortSwitch  DataPortOrder=Zero-based contiguous  Inputs=2  zeroidx=on  OutDataTypeStr=uint8  SampleTime=1  SaturateOnIntegerOverflow=off  InputSameDT=off
  emi_172_bypass : UnitDelay  InitialCondition="fi(0,0,8,0,\"hex\",\"00\")"  SampleTime=1
  emi_172 : Outport  SampleTime=1  InitialOutput=0
  wires:
  Action Port/1 -> cfblk21_out1bypassMux/1
  emi_171/1 -> cfblk21/1
  cfblk21/1 -> cfblk21_out1bypassMux/3
  cfblk21_out1bypassMux/1 -> emi_172_bypass/1, emi_172/1
  emi_172_bypass/1 -> cfblk21_out1bypassMux/2
  cfblk21_const_val/1 -> cfblk21/2

== system gm_sampleModel61442_pp_12_1_sub/Subsystem/cfblk25_inst ==
  in1 : Inport  OutDataTypeStr=uint8  SampleTime=1
  in2 : Inport  Port=2  OutDataTypeStr=uint8  SampleTime=1
  mul_cfblk25_dotp_mulcomp : Product  Inputs=**  OutDataTypeStr=uint8  SampleTime=1
  out1 : Outport  OutDataTypeStr=uint8  SampleTime=1
  wires:
  in1/1 -> mul_cfblk25_dotp_mulcomp/1
  in2/1 -> mul_cfblk25_dotp_mulcomp/2
  mul_cfblk25_dotp_mulcomp/1 -> out1/1

== system gm_sampleModel61442_pp_12_1_sub/Subsystem/cfblk28 ==
  emi_195 : Inport  OutDataTypeStr=uint8  PortDimensions=1  SampleTime=1
  Action Port : Inport  Port=2  OutDataTypeStr=boolean  SampleTime=1
  cfblk28 : Subsystem  mask(Real World Value Increment){}
      mask help: Simulink:masks:RealWorldValueIncrement_MD
      mask Display: disp('V++')
  cfblk28_out1bypassMux : MultiPortSwitch  DataPortOrder=Zero-based contiguous  Inputs=2  zeroidx=on  OutDataTypeStr=uint8  SampleTime=1  SaturateOnIntegerOverflow=off  InputSameDT=off
  emi_196_bypass : UnitDelay  InitialCondition="fi(0,0,8,0,\"hex\",\"00\")"  SampleTime=1
  emi_196 : Outport  SampleTime=1  InitialOutput=0
  wires:
  Action Port/1 -> cfblk28_out1bypassMux/1
  emi_195/1 -> cfblk28/1(u)
  cfblk28/1(y) -> cfblk28_out1bypassMux/3
  cfblk28_out1bypassMux/1 -> emi_196_bypass/1, emi_196/1
  emi_196_bypass/1 -> cfblk28_out1bypassMux/2

== system gm_sampleModel61442_pp_12_1_sub/Subsystem/cfblk3 ==
  emi_219 : Inport  OutDataTypeStr=uint8  PortDimensions=1  SampleTime=1
  Action Port : Inport  Port=2  OutDataTypeStr=boolean  SampleTime=1
  cfblk3 : Subsystem  mask(Detect Change){vinit=double(0), InputProcessing=Elements as channels (sample based), OutDataTypeStr=uint8}
      mask prompts: vinit "Simulink:masks:InitialCondition_MP"; InputProcessing "Simulink:masks:InputProcessing_MP"; OutDataTypeStr "Simulink:masks:OutputDataType_MP"
      mask help: Simulink:masks:DetectChange_MD
      mask TypeOptions InputProcessing: Simulink:masks:ColumnsAsChannelsFrameBased | Simulink:masks:ElementsAsChannelsSampleBased
      mask TypeOptions OutDataTypeStr: Simulink:masks:uint8 | Simulink:masks:boolean
      mask Display: fprintf('U ~= U/z')
  cfblk3_out1bypassMux : MultiPortSwitch  DataPortOrder=Zero-based contiguous  Inputs=2  zeroidx=on  OutDataTypeStr=uint8  SampleTime=1  SaturateOnIntegerOverflow=off  InputSameDT=off
  emi_220_bypass : UnitDelay  InitialCondition="fi(0,0,8,0,\"hex\",\"00\")"  SampleTime=1
  emi_220 : Outport  SampleTime=1  InitialOutput=0
  wires:
  Action Port/1 -> cfblk3_out1bypassMux/1, cfblk3/2(Action Port_out2)
  emi_219/1 -> cfblk3/1(U)
  cfblk3/1(Y) -> cfblk3_out1bypassMux/3
  cfblk3_out1bypassMux/1 -> emi_220_bypass/1, emi_220/1
  emi_220_bypass/1 -> cfblk3_out1bypassMux/2

== system gm_sampleModel61442_pp_12_1_sub/Subsystem/cfblk31 ==
  emi_227 : Inport  OutDataTypeStr=uint8  PortDimensions=1  SampleTime=1
  Action Port : Inport  Port=2  OutDataTypeStr=boolean  SampleTime=1
  cfblk31 : Gain  Gain="fi(0,0,8,7,\"hex\",\"80\")"  ParamDataTypeStr=fixdt(0, 8, 7)  OutDataTypeStr=fixdt(0, 16, 7)  SampleTime=1
  cfblk31_out1bypassMux : MultiPortSwitch  DataPortOrder=Zero-based contiguous  Inputs=2  zeroidx=on  OutDataTypeStr=fixdt(0, 16, 7)  SampleTime=1  SaturateOnIntegerOverflow=off  InputSameDT=off
  emi_228_bypass : UnitDelay  InitialCondition="fi(0,0,16,7,\"hex\",\"0000\")"  SampleTime=1
  emi_228 : Outport  SampleTime=1  InitialOutput=0
  wires:
  Action Port/1 -> cfblk31_out1bypassMux/1
  emi_227/1 -> cfblk31/1
  cfblk31/1 -> cfblk31_out1bypassMux/3
  cfblk31_out1bypassMux/1 -> emi_228_bypass/1, emi_228/1
  emi_228_bypass/1 -> cfblk31_out1bypassMux/2

== system gm_sampleModel61442_pp_12_1_sub/Subsystem/cfblk32 ==
  u : Inport  OutDataTypeStr=uint8  SampleTime=1
  FixPt Constant : Constant  DisableCoverage=on  OutDataTypeStr=Inherit: Inherit via back propagation  SampleTime=-1
  FixPt Data Type Duplicate : DataTypeDuplicate  DisableCoverage=on  NumInputPorts=3
  FixPt Sum1 : Sum  OutDataTypeStr=Inherit: Inherit via back propagation  InputSameDT=on  LockScale=on
  y : Outport  SampleTime=1
  wires:
  u/1 -> FixPt Sum1/1, FixPt Data Type Duplicate/2
  FixPt Constant/1 -> FixPt Sum1/2, FixPt Data Type Duplicate/3
  FixPt Sum1/1 -> FixPt Data Type Duplicate/1, y/1

== system gm_sampleModel61442_pp_12_1_sub/Subsystem/cfblk47_inst ==
  in1 : Inport  OutDataTypeStr=uint8  SampleTime=1
  in2 : Inport  Port=2  OutDataTypeStr=uint8  SampleTime=1
  mul_cfblk47_dotp_mulcomp : Product  Inputs=**  OutDataTypeStr=uint8  SampleTime=1
  out1 : Outport  OutDataTypeStr=uint8  SampleTime=1
  wires:
  in1/1 -> mul_cfblk47_dotp_mulcomp/1
  in2/1 -> mul_cfblk47_dotp_mulcomp/2
  mul_cfblk47_dotp_mulcomp/1 -> out1/1

== system gm_sampleModel61442_pp_12_1_sub/Subsystem/cfblk48 ==
  emi_139 : Inport  OutDataTypeStr=uint8  PortDimensions=1  SampleTime=1
  Action Port : Inport  Port=2  OutDataTypeStr=boolean  SampleTime=1
  cfblk48 : Abs  SampleTime=1  OutDataTypeStr=uint8  SaturateOnIntegerOverflow=off
  cfblk48_out1bypassMux : MultiPortSwitch  DataPortOrder=Zero-based contiguous  Inputs=2  zeroidx=on  OutDataTypeStr=uint8  SampleTime=1  SaturateOnIntegerOverflow=off  InputSameDT=off
  emi_140_bypass : UnitDelay  InitialCondition="fi(0,0,8,0,\"hex\",\"00\")"  SampleTime=1
  emi_140 : Outport  SampleTime=1  InitialOutput=0
  wires:
  Action Port/1 -> cfblk48_out1bypassMux/1
  emi_139/1 -> cfblk48/1
  cfblk48/1 -> cfblk48_out1bypassMux/3
  cfblk48_out1bypassMux/1 -> emi_140_bypass/1, emi_140/1
  emi_140_bypass/1 -> cfblk48_out1bypassMux/2

== system gm_sampleModel61442_pp_12_1_sub/Subsystem/cfblk52_inst ==
  in1 : Inport  OutDataTypeStr=uint8  SampleTime=1
  in2 : Inport  Port=2  OutDataTypeStr=uint8  SampleTime=1
  mul_cfblk52_dotp_mulcomp : Product  Inputs=**  OutDataTypeStr=uint8  SampleTime=1
  out1 : Outport  OutDataTypeStr=uint8  SampleTime=1
  wires:
  in1/1 -> mul_cfblk52_dotp_mulcomp/1
  in2/1 -> mul_cfblk52_dotp_mulcomp/2
  mul_cfblk52_dotp_mulcomp/1 -> out1/1

== system gm_sampleModel61442_pp_12_1_sub/Subsystem/cfblk54_inst ==
  in1 : Inport  OutDataTypeStr=uint8  SampleTime=1
  in2 : Inport  Port=2  OutDataTypeStr=uint8  SampleTime=1
  mul_cfblk54_dotp_mulcomp : Product  Inputs=**  OutDataTypeStr=uint8  SampleTime=1
  out1 : Outport  OutDataTypeStr=uint8  SampleTime=1
  wires:
  in1/1 -> mul_cfblk54_dotp_mulcomp/1
  in2/1 -> mul_cfblk54_dotp_mulcomp/2
  mul_cfblk54_dotp_mulcomp/1 -> out1/1
